simulink model "MaxPID_E_06_Modelisation_Comportement_Sujet"  (R2024b)
settings: Solver=VariableStepAuto  StartTime=0.0  StopTime=1  RelTol=1e-3
InitFcn:
  | run('parametres.m')
values from neighbouring files (symbols this model uses):
  Imax = 4.3    [parametres.m]
  K_codeur = 8192/360    (= 22.7555555556)    [parametres.m]
  K_meca = 1/110    (= 0.00909090909091)    [parametres.m]
  KD_p = 25000    [parametres.m]
  KI_p = 4800    [parametres.m]
  KP_p = 5600    [parametres.m]
  t_acc = theta_p / theta_pp    (= 0.277777777778)    [parametres.m]
  theta_p = 2.5    [parametres.m]
libraries: simulink x4
settings Model: Creator=xpess  LastModifiedBy=xpess
settings RTWCC: GPUComputeCapability=3.5

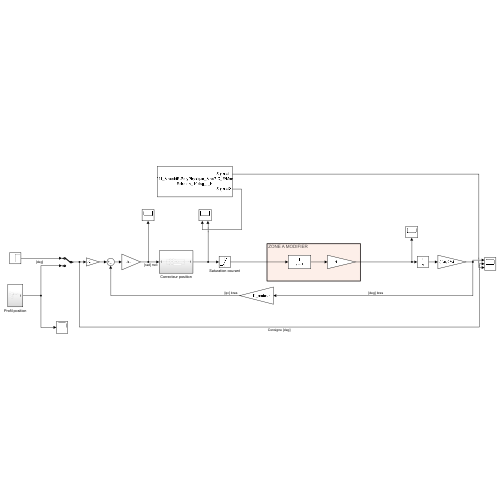
[thumbnail: Simulink's stored preview of the top-level diagram]
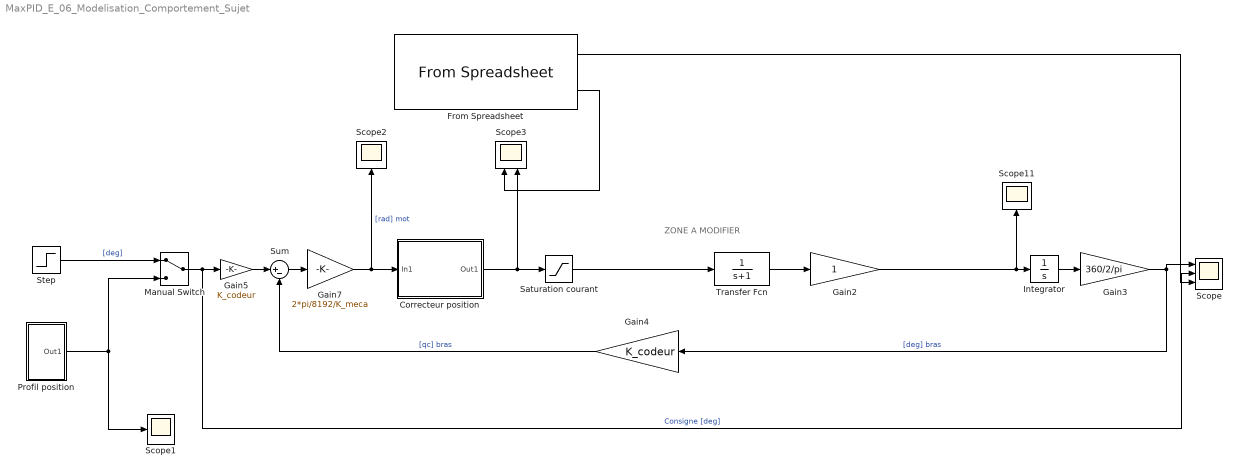
== system MaxPID_E_06_Modelisation_Comportement_Sujet ==
  note: ZONE A MODIFIER
  Correcteur position : Subsystem
  From Spreadsheet : FromSpreadsheet  FileName=C:\GitHub\TP_Documents_PSI\11_MaxpidE\PolyPhysique_MaxPID_E\Mesures\Echelon_10deg_I_H.xlsx  SheetName=Echelon_10deg_I_H  Range=A2:C103
  Gain2 : Gain
  Gain3 : Gain  Gain=360/2/pi
  Gain4 : Gain  Gain=K_codeur
  Gain5 : Gain  Gain=K_codeur
  Gain7 : Gain  Gain=2*pi/8192/K_meca
  Integrator : Integrator
  Manual Switch : ManualSwitch
  Profil position : Subsystem
  Saturation courant : Saturate  UpperLimit=Imax  LowerLimit=-Imax
  Scope : Scope  NumInputPorts=3
  Scope1 : Scope
  Scope11 : Scope
  Scope2 : Scope
  Scope3 : Scope  NumInputPorts=2
  Step : Step  Time=0  After=60  SampleTime=0
  Sum : Sum  Inputs=|+-
  Transfer Fcn : TransferFcn  Denominator=[1 1]
  wires:
  Sum/1 -> Gain7/1
  Correcteur position/1(Out1) -> Saturation courant/1, Scope3/2
  Saturation courant/1 -> Transfer Fcn/1
  Integrator/1 -> Gain3/1
  Gain3/1 -> Scope/1, Gain4/1  "[deg] bras"
  Gain5/1 -> Sum/1
  Step/1 -> Manual Switch/1  "[deg]"
  Profil position/1(Out1) -> Manual Switch/2, Scope1/1
  Manual Switch/1 -> Scope/2, Gain5/1  "Consigne [deg]"
  Gain2/1 -> Scope11/1, Integrator/1
  Gain7/1 -> Scope2/1, Correcteur position/1(In1)  "[rad] mot"
  From Spreadsheet/1 -> Scope/3
  Transfer Fcn/1 -> Gain2/1
  Gain4/1 -> Sum/2  "[qc] bras"
  From Spreadsheet/2 -> Scope3/1

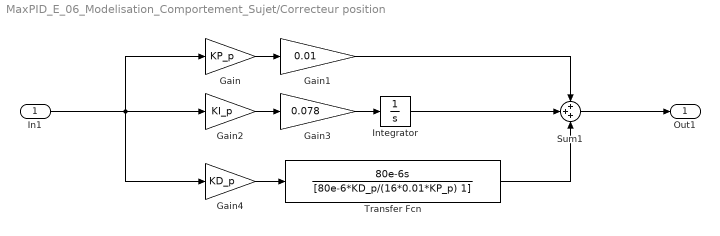
== system MaxPID_E_06_Modelisation_Comportement_Sujet/Correcteur position ==
  In1 : Inport
  Gain : Gain  Gain=KP_p
  Gain1 : Gain  Gain=0.01
  Gain2 : Gain  Gain=KI_p
  Gain3 : Gain  Gain=0.078
  Gain4 : Gain  Gain=KD_p
  Integrator : Integrator
  Sum1 : Sum  Inputs=+++
  Transfer Fcn : TransferFcn  Numerator=[80e-6 0]  Denominator=[80e-6*KD_p/(16*0.01*KP_p) 1]
  Out1 : Outport
  wires:
  Transfer Fcn/1 -> Sum1/3
  Gain/1 -> Gain1/1
  In1/1 -> Gain/1, Gain4/1, Gain2/1
  Gain2/1 -> Gain3/1
  Integrator/1 -> Sum1/2
  Gain4/1 -> Transfer Fcn/1
  Gain3/1 -> Integrator/1
  Sum1/1 -> Out1/1
  Gain1/1 -> Sum1/1

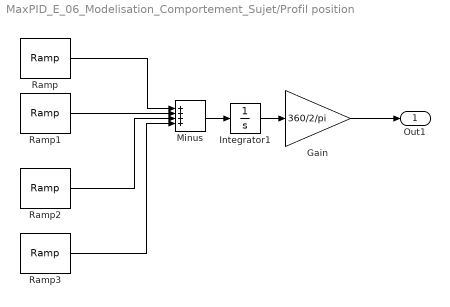
== system MaxPID_E_06_Modelisation_Comportement_Sujet/Profil position ==
  Gain : Gain  Gain=360/2/pi
  Integrator1 : Integrator
  Minus : Sum  Inputs=++++
  Ramp : simulink/Sources/Ramp  slope=theta_p/t_acc  start=t0  InitialOutput=0
  Ramp1 : simulink/Sources/Ramp  slope=-theta_p/t_acc  start=t1  InitialOutput=0
  Ramp2 : simulink/Sources/Ramp  slope=-theta_p/t_acc  start=t2  InitialOutput=0
  Ramp3 : simulink/Sources/Ramp  slope=theta_p/t_acc  start=t3  InitialOutput=0
  Out1 : Outport
  wires:
  Ramp/1 -> Minus/1
  Integrator1/1 -> Gain/1
  Ramp3/1 -> Minus/4
  Ramp1/1 -> Minus/2
  Ramp2/1 -> Minus/3
  Minus/1 -> Integrator1/1
  Gain/1 -> Out1/1
